simulink library "SimscapeCustomComponents_lib"  (R2025b)
settings: Solver=VariableStepAuto  StartTime=0.0  StopTime=10.0  RelTol=1e-3
undefined symbols (not defined in the file or in its folder): base, baseVdc, capacity, DiscIntNeverNeededParam, ee_sli_rtmsupport, filterInductance, freqeuncy, frequency, gcbh, gflInverter, gfmInverter, iMaxPU, Inertia, initialSOC, plantRating, solar, Ts, ups, Vac, windSystem, windTurbine
libraries: fl_lib x397, nesl_utility x171, eeGeneralControl x85, ee_lib x82, simulink x72, datacenter_lib x68, eeTransforms x38, slpidlib x24, buildingEnergy_lib x20, SimscapeFluids_lib x17, eeSinusoidalMeasurementV2 x8, eePwmGenerator x8
(part 8 of 24)

== system SimscapeCustomComponents_lib/Datacenter/Assemblies/Air Cooled PDU Assembly/PDU Racks ==
  PS Product : fl_lib/Physical Signals/Functions/PS Product
  Server Tray : Subsystem  mask{nGPU=nGPU, gpuTDPperDie=gpuTDPperDie, gpuIdlePower=gpuIdlePower, gpuHBMpower=gpuHBMpower, gpuExponent=gpuExponent, gpuHBMutil=gpuHBMutil, gpuLeakage=gpuLeakage, gpuNominalDieT=gpuNominalDieT, gpuDieThermalC=gpuDieThermalC, gpuHeatSinkR=gpuHeatSinkR, gpuSurfArea=gpuSurfArea, gpuAmbientR=gpuAmbientR, nCPU=nCPU, cpuTDPperSocket=cpuTDPperSocket, cpuIdlePower=cpuIdlePower, cpuExponent=cpuExponent, cpuLeakage=cpuLeakage, cpuNominalDieT=cpuNominalDieT, cpuDieThermalC=cpuDieThermalC, cpuHeatSinkR=cpuHeatSinkR, cpuSurfArea=cpuSurfArea, cpuAmbientR=cpuAmbientR, trayMass=trayMass, trayCp=trayCp, trayThermalR=trayThermalR, initialT=initialT, htc=htc}
      mask prompts: nGPU "Number of GPU (-)"; gpuTDPperDie "GPU TDP per die (W)"; gpuIdlePower "GPU idle power (W)"; gpuHBMpower "HBM power per GPU (W)"; gpuExponent "GPU power utilization exponent (-)"; gpuHBMutil "HBM utilization as fraction of compute utilization (-)"; gpuLeakage "Leakage increase per K above nominal temperature (W/K)"; gpuNominalDieT "Nominal die temperature at TDP (K)"; gpuDieThermalC "GPU die thermal capacitance (J/K)"; gpuHeatSinkR "GPU die-heat-sink thermal resistance (K/W)"; gpuSurfArea "Surface area per die for ambient heat transfer (m^2)"; gpuAmbientR "GPU die-ambient thermal resistance (K/W)"; nCPU "Number of CPU (-)"; cpuTDPperSocket "CPU TDP per socket (W)"; cpuIdlePower "CPU idle power per socket (W)"; cpuExponent "CPU power utilization exponent (-)"; cpuLeakage "Leakage increase per K above nominal temperature (W/K)"; cpuNominalDieT "Nominal die temperature at TDP (K)"; cpuDieThermalC "CPU die thermal capacitance (J/K)"; cpuHeatSinkR "CPU die-heat-sink thermal resistance (K/W)"; cpuSurfArea "Surface area per die for ambient heat transfer (m^2)"; cpuAmbientR "CPU die-ambient thermal resistance (K/W)"; trayMass "Tray mass (kg)"; trayCp "Tray specific heat capacity (J/kg*K)"; trayThermalR "Tray to external thermal resistance (K/W)"; initialT "Initial temperature (K)"; htc "Heat transfer coefficient to ambient (W/m^2.K)"
      settings: CopyFcn=set_param(gcbh,'LinkStatus','none');  PortSchema="{\"entries\":[{\"content\":{\"sides\":[{\"content\":{\"connectorIds\":[\"LConn1\",\"LConn2\",\"LConn3\"]},\"type\":\"ConnectorPlacement.EquallySpacedRectSide\",\"uuid\":\"893f21b9-92d6-433a-96e5-f8193a696c29\"},{\"content\":{\"connectorIds\":[\"RConn1\",\"RConn2\",\"RConn3\"],\"side\":\"RIGHT\"},\"type\":\"ConnectorPlacement.EquallySpacedRectSide\",\"uuid\":\"efd10409-70d8-4a6a-97a2-13f0e6f538e3\"},{\"content\":{\"side\":\"TOP\"},\"type\":\"ConnectorPlacement.EquallySpacedRectSide\",\"uuid\":\"8c9765cd-90e6-46de-916c-606bbb93143e\"},{\"content\":{\"connectorIds\":[\"RConn4\"],\"side\":\"BOTTOM\"},\"type\":\"ConnectorPlacement.EquallySpacedRectSide\",\"uuid\":\"9656b44e-d582-43b0-a7fe-c629821d6c27\"}]},\"type\":\"ConnectorPlacement.EquallySpacedConnector\",\"uuid\":\"add7a682-eb4b-4f46-a5b9-e161ccf96de5\"}],\"packageUris\":[\"http://schema.mathworks.com/mf0/Connector/R2020b\"],\"version\":\"1.0\"}"
      mask Help: web("DocumentationServerTray.html")
      mask DialogControl Container6 Prompt: GPU
      mask DialogControl Container7 Prompt: CPU
      mask DialogControl Container9 Prompt: IT Tray
      mask DialogControl Container8 Prompt: Initial Conditions
      mask Display: image('icon_serverPlate.png');
  TMamb : datacenter_lib/Thermal Multiplier
      settings: InternalSimscapePortConfiguration="{\"Bottom\":[],\"Left\":[{\"id\":\"A\",\"label\":\"A\",\"type\":\"foundation.thermal.thermal\"}],\"Right\":[{\"id\":\"B\",\"label\":\"B\",\"type\":\"foundation.thermal.thermal\"}],\"Top\":[{\"id\":\"Na\",\"label\":\"Na\",\"type\":\"input\"},{\"id\":\"Nb\",\"label\":\"Nb\",\"type\":\"input\"}]}"
  TMcdu : datacenter_lib/Thermal Multiplier
      settings: InternalSimscapePortConfiguration="{\"Bottom\":[],\"Left\":[{\"id\":\"A\",\"label\":\"A\",\"type\":\"foundation.thermal.thermal\"}],\"Right\":[{\"id\":\"B\",\"label\":\"B\",\"type\":\"foundation.thermal.thermal\"}],\"Top\":[{\"id\":\"Na\",\"label\":\"Na\",\"type\":\"input\"},{\"id\":\"Nb\",\"label\":\"Nb\",\"type\":\"input\"}]}"
  nTraysXnRacks : fl_lib/Physical Signals/Sources/PS Constant  constant=nTrays*nRacks
  one : fl_lib/Physical Signals/Sources/PS Constant  constant=1
  U_gpu : PMIOPort  Side=Left
  U_cpu : PMIOPort  Port=2  Side=Left
  Ha : PMIOPort  Port=3  Side=Left
  P : PMIOPort  Port=4  Side=Right
  T_gpu : PMIOPort  Port=5  Side=Right
  T_cpu : PMIOPort  Port=6  Side=Right
  Hc : PMIOPort  Port=7  Side=Right
  connections:
  PS Product/RConn1 -- P/RConn1
  Server Tray/RConn1 -- PS Product/LConn2
  TMamb/LConn3 -- TMcdu/LConn2 -- PS Product/LConn1 -- nTraysXnRacks/RConn1
  Server Tray/LConn3 -- TMamb/RConn1
  Server Tray/RConn4 -- TMcdu/LConn1
  TMamb/LConn2 -- TMcdu/LConn3 -- one/RConn1
  Server Tray/RConn3 -- T_cpu/RConn1
  Server Tray/LConn2 -- U_cpu/RConn1
  TMcdu/RConn1 -- Hc/RConn1
  Server Tray/RConn2 -- T_gpu/RConn1
  TMamb/LConn1 -- Ha/RConn1
  Server Tray/LConn1 -- U_gpu/RConn1

== system SimscapeCustomComponents_lib/Datacenter/Assemblies/Air Cooled PDU Assembly/Rack Air Cooling ==
  Flowrate vs Eff : fl_lib/Physical Signals/Lookup Tables/PS Lookup Table (1D)  x=flowVec m^3/s  f=fanEffVec  interp_method=simscape.enum.interpolation.linear  extrap_method=simscape.enum.extrapolation.nearest
  Flowrate vs Pressure Drop : fl_lib/Physical Signals/Lookup Tables/PS Lookup Table (1D)  x=flowVec m^3/s  f=prDropVec Pa  interp_method=simscape.enum.interpolation.linear  extrap_method=simscape.enum.extrapolation.nearest
  MaxFlowrate : fl_lib/Physical Signals/Functions/PS Gain  gain=max(flowVec) m^3/s
  PS Divide : fl_lib/Physical Signals/Functions/PS Divide
  PS Product : fl_lib/Physical Signals/Functions/PS Product
  PS Product1 : fl_lib/Physical Signals/Functions/PS Product
  PS Saturation : fl_lib/Physical Signals/Nonlinear Operators/PS Saturation  upper_limit=1  lower_limit=0  ZeroCross=true
  Q : Subsystem
  dT : Subsystem
      settings: PortSchema="{\"entries\":[{\"content\":{\"sides\":[{\"content\":{\"connectorIds\":[\"LConn1\"]},\"type\":\"ConnectorPlacement.EquallySpacedRectSide\",\"uuid\":\"24179a54-9ef9-408d-b9e3-71fcbe48c3e7\"},{\"content\":{\"connectorIds\":[\"RConn1\"],\"side\":\"RIGHT\"},\"type\":\"ConnectorPlacement.EquallySpacedRectSide\",\"uuid\":\"9ef8b705-2d29-4693-9aa8-2fb03fb72ba0\"},{\"content\":{\"side\":\"TOP\"},\"type\":\"ConnectorPlacement.EquallySpacedRectSide\",\"uuid\":\"67fd6558-0b74-41b6-9065-c50d20bb7de5\"},{\"content\":{\"connectorIds\":[\"RConn2\"],\"side\":\"BOTTOM\"},\"type\":\"ConnectorPlacement.EquallySpacedRectSide\",\"uuid\":\"dead0843-c913-4c5f-8840-2a92db603c86\"}]},\"type\":\"ConnectorPlacement.EquallySpacedConnector\",\"uuid\":\"734a32c8-d564-4672-86f6-d3d1b9b4eb6d\"}],\"packageUris\":[\"http://schema.mathworks.com/mf0/Connector/R2020b\"],\"version\":\"1.0\"}"
  m_dot_Cp : Subsystem
      settings: PortSchema="{\"entries\":[{\"content\":{\"sides\":[{\"content\":{},\"type\":\"ConnectorPlacement.EquallySpacedRectSide\",\"uuid\":\"30dae9bf-ed85-460d-bbc0-602f54b59459\"},{\"content\":{\"side\":\"RIGHT\"},\"type\":\"ConnectorPlacement.EquallySpacedRectSide\",\"uuid\":\"05907a20-db7b-437b-af9c-28a9e12dbb0f\"},{\"content\":{\"connectorIds\":[\"LConn1\"],\"side\":\"TOP\"},\"type\":\"ConnectorPlacement.EquallySpacedRectSide\",\"uuid\":\"1394250d-0f3a-4d32-aa79-d5be723ed221\"},{\"content\":{\"connectorIds\":[\"RConn1\"],\"side\":\"BOTTOM\"},\"type\":\"ConnectorPlacement.EquallySpacedRectSide\",\"uuid\":\"8d71629e-6ed3-4a45-8875-f0ad6e4187c2\"}]},\"type\":\"ConnectorPlacement.EquallySpacedConnector\",\"uuid\":\"77e9989b-961e-42ca-a28b-c98959ddb965\"}],\"packageUris\":[\"http://schema.mathworks.com/mf0/Connector/R2020b\"],\"version\":\"1.0\"}"
  numFans : fl_lib/Physical Signals/Sources/PS Constant  constant=nFans
  C : PMIOPort  Side=Left
  S : PMIOPort  Port=2  Side=Left
  H : PMIOPort  Port=3  Side=Right
  P : PMIOPort  Port=4  Side=Right
  connections:
  m_dot_Cp/LConn1 -- Q/LConn2
  Q/LConn1 -- dT/RConn2
  dT/LConn1 -- C/RConn1
  H/RConn1 -- dT/RConn1 -- Q/RConn1
  PS Product/LConn1 -- Flowrate vs Pressure Drop/RConn1
  numFans/RConn1 -- PS Product1/LConn1
  PS Saturation/RConn1 -- MaxFlowrate/LConn1
  PS Divide/RConn1 -- P/RConn1
  PS Divide/LConn2 -- Flowrate vs Eff/RConn1
  PS Product1/RConn1 -- PS Divide/LConn1
  PS Saturation/LConn1 -- S/RConn1
  PS Product1/LConn2 -- PS Product/RConn1
  m_dot_Cp/RConn1 -- MaxFlowrate/RConn1 -- Flowrate vs Pressure Drop/LConn1 -- PS Product/LConn2 -- Flowrate vs Eff/LConn1

== system SimscapeCustomComponents_lib/Datacenter/Assemblies/PDU + CDU Assembly (LUT)/CDU (LUT) ==
  Capacity vs. Flowrate : fl_lib/Physical Signals/Lookup Tables/PS Lookup Table (1D)  x=flowrate_vec m^3/s  f=capacity_vec W  interp_method=simscape.enum.interpolation.linear  extrap_method=simscape.enum.extrapolation.nearest
  Controlled Heat Flow Rate Source : fl_lib/Thermal/Thermal Sources/Controlled Heat Flow Rate Source
  Electric Power : fl_lib/Physical Signals/Functions/PS Divide
  PS Product : fl_lib/Physical Signals/Functions/PS Product
  PS Product1 : fl_lib/Physical Signals/Functions/PS Product
  Pressure Drop vs. Num Pump & Flowrate : fl_lib/Physical Signals/Lookup Tables/PS Lookup Table (2D)  x1=flowrate_vec m^3/s  x2=1:numPump  f=prDrop_mat Pa  interp_method=simscape.enum.interpolation.linear  extrap_method=simscape.enum.extrapolation.nearest
  Pump Eff. vs. Flowrate : fl_lib/Physical Signals/Lookup Tables/PS Lookup Table (1D)  x=flowrate_vec m^3/s  f=effPump_vec  interp_method=simscape.enum.interpolation.linear  extrap_method=simscape.enum.extrapolation.nearest
  Thermal Reference : fl_lib/Thermal/Thermal Elements/Thermal Reference
  flowrate : Subsystem
  S : PMIOPort  Side=Left
  N : PMIOPort  Port=2  Side=Left
  H : PMIOPort  Port=3  Side=Left
  P : PMIOPort  Port=4  Side=Right
  Q : PMIOPort  Port=5  Side=Right
  connections:
  S/RConn1 -- flowrate/LConn1
  Capacity vs. Flowrate/LConn1 -- flowrate/RConn1 -- PS Product/LConn2 -- Pump Eff. vs. Flowrate/LConn1 -- Pressure Drop vs. Num Pump & Flowrate/LConn1
  Controlled Heat Flow Rate Source/RConn1 -- Q/RConn1 -- PS Product1/RConn1
  Capacity vs. Flowrate/RConn1 -- PS Product1/LConn1
  Controlled Heat Flow Rate Source/RConn2 -- H/RConn1
  Electric Power/LConn1 -- PS Product/RConn1
  Electric Power/RConn1 -- P/RConn1
  PS Product/LConn1 -- Pressure Drop vs. Num Pump & Flowrate/RConn1
  N/RConn1 -- Pressure Drop vs. Num Pump & Flowrate/LConn2 -- PS Product1/LConn2
  Controlled Heat Flow Rate Source/LConn1 -- Thermal Reference/LConn1
  Electric Power/LConn2 -- Pump Eff. vs. Flowrate/RConn1

== system SimscapeCustomComponents_lib/Datacenter/Assemblies/PDU + CDU Assembly (LUT)/PDU Racks ==
  PS Product : fl_lib/Physical Signals/Functions/PS Product
  Server Tray : Subsystem  mask{nGPU=nGPU, gpuTDPperDie=gpuTDPperDie, gpuIdlePower=gpuIdlePower, gpuHBMpower=gpuHBMpower, gpuExponent=gpuExponent, gpuHBMutil=gpuHBMutil, gpuLeakage=gpuLeakage, gpuNominalDieT=gpuLeakage, gpuDieThermalC=gpuDieThermalC, gpuHeatSinkR=gpuHeatSinkR, gpuSurfArea=gpuSurfArea, gpuAmbientR=gpuAmbientR, nCPU=nCPU, cpuTDPperSocket=cpuTDPperSocket, cpuIdlePower=cpuIdlePower, cpuExponent=cpuExponent, cpuLeakage=cpuLeakage, cpuNominalDieT=cpuNominalDieT, cpuDieThermalC=cpuDieThermalC, cpuHeatSinkR=cpuHeatSinkR, cpuSurfArea=cpuSurfArea, cpuAmbientR=cpuAmbientR, trayMass=trayMass, trayCp=trayCp, trayThermalR=trayThermalR, initialT=initialT, htc=htc}
      mask prompts: nGPU "Number of GPU (-)"; gpuTDPperDie "GPU TDP per die (W)"; gpuIdlePower "GPU idle power (W)"; gpuHBMpower "HBM power per GPU (W)"; gpuExponent "GPU power utilization exponent (-)"; gpuHBMutil "HBM utilization as fraction of compute utilization (-)"; gpuLeakage "Leakage increase per K above nominal temperature (W/K)"; gpuNominalDieT "Nominal die temperature at TDP (K)"; gpuDieThermalC "GPU die thermal capacitance (J/K)"; gpuHeatSinkR "GPU die-heat-sink thermal resistance (K/W)"; gpuSurfArea "Surface area per die for ambient heat transfer (m^2)"; gpuAmbientR "GPU die-ambient thermal resistance (K/W)"; nCPU "Number of CPU (-)"; cpuTDPperSocket "CPU TDP per socket (W)"; cpuIdlePower "CPU idle power per socket (W)"; cpuExponent "CPU power utilization exponent (-)"; cpuLeakage "Leakage increase per K above nominal temperature (W/K)"; cpuNominalDieT "Nominal die temperature at TDP (K)"; cpuDieThermalC "CPU die thermal capacitance (J/K)"; cpuHeatSinkR "CPU die-heat-sink thermal resistance (K/W)"; cpuSurfArea "Surface area per die for ambient heat transfer (m^2)"; cpuAmbientR "CPU die-ambient thermal resistance (K/W)"; trayMass "Tray mass (kg)"; trayCp "Tray specific heat capacity (J/kg*K)"; trayThermalR "Tray to external thermal resistance (K/W)"; initialT "Initial temperature (K)"; htc "Heat transfer coefficient to ambient (W/m^2.K)"
      settings: CopyFcn=set_param(gcbh,'LinkStatus','none');  PortSchema="{\"entries\":[{\"content\":{\"sides\":[{\"content\":{\"connectorIds\":[\"LConn1\",\"LConn2\",\"LConn3\"]},\"type\":\"ConnectorPlacement.EquallySpacedRectSide\",\"uuid\":\"893f21b9-92d6-433a-96e5-f8193a696c29\"},{\"content\":{\"connectorIds\":[\"RConn1\",\"RConn2\",\"RConn3\"],\"side\":\"RIGHT\"},\"type\":\"ConnectorPlacement.EquallySpacedRectSide\",\"uuid\":\"efd10409-70d8-4a6a-97a2-13f0e6f538e3\"},{\"content\":{\"side\":\"TOP\"},\"type\":\"ConnectorPlacement.EquallySpacedRectSide\",\"uuid\":\"8c9765cd-90e6-46de-916c-606bbb93143e\"},{\"content\":{\"connectorIds\":[\"RConn4\"],\"side\":\"BOTTOM\"},\"type\":\"ConnectorPlacement.EquallySpacedRectSide\",\"uuid\":\"9656b44e-d582-43b0-a7fe-c629821d6c27\"}]},\"type\":\"ConnectorPlacement.EquallySpacedConnector\",\"uuid\":\"add7a682-eb4b-4f46-a5b9-e161ccf96de5\"}],\"packageUris\":[\"http://schema.mathworks.com/mf0/Connector/R2020b\"],\"version\":\"1.0\"}"
      mask Help: web("DocumentationServerTray.html")
      mask DialogControl Container6 Prompt: GPU
      mask DialogControl Container7 Prompt: CPU
      mask DialogControl Container9 Prompt: IT Tray
      mask DialogControl Container8 Prompt: Initial Conditions
      mask Display: image('icon_serverPlate.png');
  TMamb : datacenter_lib/Thermal Multiplier
      settings: InternalSimscapePortConfiguration="{\"Bottom\":[],\"Left\":[{\"id\":\"A\",\"label\":\"A\",\"type\":\"foundation.thermal.thermal\"}],\"Right\":[{\"id\":\"B\",\"label\":\"B\",\"type\":\"foundation.thermal.thermal\"}],\"Top\":[{\"id\":\"Na\",\"label\":\"Na\",\"type\":\"input\"},{\"id\":\"Nb\",\"label\":\"Nb\",\"type\":\"input\"}]}"
  TMcdu : datacenter_lib/Thermal Multiplier
      settings: InternalSimscapePortConfiguration="{\"Bottom\":[],\"Left\":[{\"id\":\"A\",\"label\":\"A\",\"type\":\"foundation.thermal.thermal\"}],\"Right\":[{\"id\":\"B\",\"label\":\"B\",\"type\":\"foundation.thermal.thermal\"}],\"Top\":[{\"id\":\"Na\",\"label\":\"Na\",\"type\":\"input\"},{\"id\":\"Nb\",\"label\":\"Nb\",\"type\":\"input\"}]}"
  nTraysXnRacks : fl_lib/Physical Signals/Sources/PS Constant  constant=nTrays*nRacks
  one : fl_lib/Physical Signals/Sources/PS Constant  constant=1
  U_gpu : PMIOPort  Side=Left
  U_cpu : PMIOPort  Port=2  Side=Left
  Ha : PMIOPort  Port=3  Side=Left
  P : PMIOPort  Port=4  Side=Right
  T_gpu : PMIOPort  Port=5  Side=Right
  T_cpu : PMIOPort  Port=6  Side=Right
  Hc : PMIOPort  Port=7  Side=Right
  connections:
  PS Product/RConn1 -- P/RConn1
  Server Tray/RConn1 -- PS Product/LConn2
  TMamb/LConn3 -- TMcdu/LConn2 -- PS Product/LConn1 -- nTraysXnRacks/RConn1
  Server Tray/LConn3 -- TMamb/RConn1
  Server Tray/RConn4 -- TMcdu/LConn1
  TMamb/LConn2 -- TMcdu/LConn3 -- one/RConn1
  Server Tray/RConn3 -- T_cpu/RConn1
  Server Tray/LConn2 -- U_cpu/RConn1
  TMcdu/RConn1 -- Hc/RConn1
  Server Tray/RConn2 -- T_gpu/RConn1
  TMamb/LConn1 -- Ha/RConn1
  Server Tray/LConn1 -- U_gpu/RConn1

== system SimscapeCustomComponents_lib/Datacenter/Assemblies/PDU + CDU Assembly (TL)/CDU (TL) ==
  CDU Pipe : fl_lib/Thermal Liquid/Elements/Pipe (TL)  length=effPipeLen m  area=intFluidPipeArea m^2  Dh=sqrt(4*intFluidPipeArea/pi) m  length_add=1e-2 m  roughness=15e-6 m  Re_lam=2000  Re_tur=4000  shape_factor=64  Nu_lam=3.66  dynamic_compressibility=true  inertia=false  p0=iniP MPa  T0=iniT K  mdot0=0 kg/s  p_nominal=0.101325 MPa  T_nominal=293.15 K
  Centrifugal Pump (TL) : SimscapeFluids_lib/Thermal Liquid/Pumps & Motors/Centrifugal Pump (TL)  pump_parameterization=fluids.thermal_liquid.pumps_motors.enum.CentrifugalPumpParameterization.Table1D  capacity_ref_nominal=45 lpm  head_ref_nominal=40 m  power_ref_nominal=0.85 kW  head_ref_max=60 m  capacity_ref_max=80 lpm  omega_ref_analytic=1770 rpm  flow_rate_1D_TLU=pumpCapacityVec m^3/s  head_1D_TLU=pumpRefHeadVec m  power_1D_TLU=pumpRefBrkPowVec kW  omega_ref_1D=pumpNominalRPM rpm  rho_ref_1D=refDensity kg/m^3  omega_threshold_factor=1e-2  flow_rate_2D_TLU=[16.67, 23.33, 30, 40, 53.33, 60] lpm  omega_2D_TLU=[2450, 2800, 3150, 3500] rpm  head_2D_TLU=[25, 32.7, 42.5, 50; 24, 31.7, 41, 49; 22.7, 30.5, 39, 47.5; 20, 28, 36, 45; 15.7, 24, 32, 40; 12.5, 21, 29.5, 37.5] m  power_2D_TLU=[.28, .38, .5, .6; .31, .41, .55, .68; .33, .44, .6, .75; .36, .48, .65, .83; .38, .53, .72, .93; .39, .55, .75, .97] kW  rho_ref_2D=998.21 kg/m^3  diameter_ratio=pumpImpellerDiaFactor  mech_orientation=fluids.thermal_liquid.pumps_motors.enum.CentrifugalPumpMechOrientation.Positive  area=intFluidPipeArea/nPumps m^2  operation_check=simscape.enum.assert.action.none
      settings: InternalSimscapePortConfiguration="{\"Bottom\":[],\"Left\":[{\"id\":\"A\",\"label\":\"A\",\"type\":\"foundation.thermal_liquid.thermal_liquid\"},{\"id\":\"B\",\"label\":\"B\",\"type\":\"foundation.thermal_liquid.thermal_liquid\"}],\"Right\":[{\"id\":\"R\",\"label\":\"R\",\"type\":\"foundation.mechanical.rotational.rotational\"},{\"id\":\"C\",\"label\":\"C\",\"type\":\"foundation.mechanical.rotational.rotational\"}],\"Top\":[]}"
  Expansion Tank : SimscapeFluids_lib/Thermal Liquid/Tanks & Accumulators/Gas-Charged Accumulator (TL)  capacity=intFluidVol m^3  dead_volume=1e-3 m^3  p_precharge_gauge=iniP MPa  k_sh=1.4  area=intFluidPipeArea m^2  stiff_coeff=1e4 MPa/m^3  damping_coeff=1e4 MPa*s/m^6  liquid_volume_specify=on  liquid_volume_priority=None  liquid_volume=5e-3 m^3  liquid_volume_nominal_specify=off  liquid_volume_nominal_value=1  liquid_volume_nominal_unit=m^3  liquid_mass_specify=off  liquid_mass_priority=None  liquid_mass=5 kg  liquid_mass_nominal_specify=off  liquid_mass_nominal_value=1  liquid_mass_nominal_unit=kg  p_I_specify=on  p_I_priority=High  p_I=4*iniP MPa  p_I_nominal_specify=off  p_I_nominal_value=1  p_I_nominal_unit=MPa  T_I_specify=on  T_I_priority=High  T_I=iniT K  T_I_nominal_specify=off  T_I_nominal_value=1  T_I_nominal_unit=K
      settings: InternalSimscapePortConfiguration="{\"Bottom\":[],\"Left\":[],\"Right\":[{\"id\":\"A\",\"label\":\"A\",\"type\":\"foundation.thermal_liquid.thermal_liquid\"},{\"id\":\"H\",\"label\":\"H\",\"type\":\"foundation.thermal.thermal\"}],\"Top\":[]}"
  Flow Multiplier : datacenter_lib/Flow Multiplier
      settings: InternalSimscapePortConfiguration="{\"Bottom\":[],\"Left\":[{\"id\":\"A\",\"label\":\"A\",\"type\":\"foundation.thermal_liquid.thermal_liquid\"}],\"Right\":[{\"id\":\"B\",\"label\":\"B\",\"type\":\"foundation.thermal_liquid.thermal_liquid\"}],\"Top\":[{\"id\":\"Na\",\"label\":\"Na\",\"type\":\"input\"},{\"id\":\"Nb\",\"label\":\"Nb\",\"type\":\"input\"}]}"
  "Flow Multiplier " : datacenter_lib/Flow Multiplier
      settings: InternalSimscapePortConfiguration="{\"Bottom\":[],\"Left\":[{\"id\":\"A\",\"label\":\"A\",\"type\":\"foundation.thermal_liquid.thermal_liquid\"}],\"Right\":[{\"id\":\"B\",\"label\":\"B\",\"type\":\"foundation.thermal_liquid.thermal_liquid\"}],\"Top\":[{\"id\":\"Na\",\"label\":\"Na\",\"type\":\"input\"},{\"id\":\"Nb\",\"label\":\"Nb\",\"type\":\"input\"}]}"
  Flow Rate Sensor (TL) : fl_lib/Thermal Liquid/Sensors/Flow Rate Sensor (TL)  mass_flow_measure=false  volumetric_flow_measure=true  energy_flow_measure=false
      settings: InternalSimscapePortConfiguration="{\"Bottom\":[],\"Left\":[{\"id\":\"A\",\"label\":\"A\",\"type\":\"foundation.thermal_liquid.thermal_liquid\"}],\"Right\":[{\"id\":\"B\",\"label\":\"B\",\"type\":\"foundation.thermal_liquid.thermal_liquid\"},{\"id\":\"V\",\"label\":\"V\",\"type\":\"output\"}],\"Top\":[]}"
  Flow Resistance (TL) : fl_lib/Thermal Liquid/Elements/Flow Resistance (TL)  delta_p_nominal=0.1*min(intFluidPrDrop) kPa  mdot_nominal=min(intFluidMdot) kg/s  area=intFluidPipeArea m^2  laminar_fraction=1e-3
  "Flow Resistance (TL) " : fl_lib/Thermal Liquid/Elements/Flow Resistance (TL)  delta_p_nominal=0.1*min(intFluidPrDrop) kPa  mdot_nominal=min(intFluidMdot) kg/s  area=intFluidPipeArea m^2  laminar_fraction=1e-3
  InternalFluid : SimscapeFluids_lib/Thermal Liquid/Utilities/Thermal Liquid Properties (TL)  fluid_list=fluids.thermal_liquid.utilities.enum.thermal_liquid_fluid_list.water  concentration_param_EG=fluids.thermal_liquid.utilities.enum.thermal_liquid_concentration.volume_fraction  concentration_param_PG=fluids.thermal_liquid.utilities.enum.thermal_liquid_concentration.volume_fraction  c_mass_SW=3.5e-3  c_mass_EG=0.1  c_mass_PG=0.1  c_mass_GL=0.1  c_vol_EG=0.1  c_vol_PG=0.1  beta_const_EG=2.1791 GPa  beta_const_PG=2.1791 GPa  beta_const_GL=2.1791 GPa  p_min_EG=0.01 MPa  p_min_PG=0.01 MPa  p_min_GL=0.01 MPa  p_max_EG=50 MPa  p_max_PG=50 MPa  p_max_GL=50 MPa  p_atm=0.101325 MPa  properties_range_check=simscape.enum.assert.action.error
  One : fl_lib/Physical Signals/Sources/PS Constant  constant=1
  PS Saturation : fl_lib/Physical Signals/Nonlinear Operators/PS Saturation  upper_limit=speedLimFactor  lower_limit=0  ZeroCross=true
  Perfect Insulator1 : fl_lib/Thermal/Thermal Elements/Perfect Insulator  T_specify=off  T_priority=None  T=293.15 K  T_nominal_specify=off  T_nominal_value=1  T_nominal_unit=K
  Pressure & Temperature Sensor (TL) : fl_lib/Thermal Liquid/Sensors/Pressure & Temperature Sensor (TL)  reference=foundation.enum.MeasurementReference.difference  pressure=true  pressure_spec=foundation.enum.PressureMeasementSpec.Absolute  temperature=false
      settings: InternalSimscapePortConfiguration="{\"Bottom\":[],\"Left\":[{\"id\":\"A\",\"label\":\"A\",\"type\":\"foundation.thermal_liquid.thermal_liquid\"}],\"Right\":[{\"id\":\"B\",\"label\":\"B\",\"type\":\"foundation.thermal_liquid.thermal_liquid\"},{\"id\":\"P\",\"label\":\"P\",\"type\":\"output\"}],\"Top\":[]}"
  Pump Efficiency : Subsystem
      settings: PortSchema="{\"entries\":[{\"content\":{\"sides\":[{\"content\":{\"connectorIds\":[\"LConn1\"]},\"type\":\"ConnectorPlacement.EquallySpacedRectSide\",\"uuid\":\"7c880f53-79d7-4fc1-b853-6a19eeb267d6\"},{\"content\":{\"connectorIds\":[\"RConn1\"],\"side\":\"RIGHT\"},\"type\":\"ConnectorPlacement.EquallySpacedRectSide\",\"uuid\":\"ee796b5d-8f71-4c2c-8982-d65c9b09dfff\"},{\"content\":{\"connectorIds\":[\"LConn2\",\"LConn3\"],\"side\":\"TOP\"},\"type\":\"ConnectorPlacement.EquallySpacedRectSide\",\"uuid\":\"11e8f51e-a30e-473a-bd43-abeec225f5c9\"}]},\"type\":\"ConnectorPlacement.EquallySpacedConnector\",\"uuid\":\"3106b96b-5b56-4bfa-809a-5c3e3f25fbb5\"}],\"packageUris\":[\"http://schema.mathworks.com/mf0/Connector/R2020b\"],\"version\":\"1.0\"}"
  Pump Nominal Rating : fl_lib/Physical Signals/Functions/PS Gain  gain=pumpNominalRPM rpm
  Specific Dissipation Heat Exchanger (TL-TL) : SimscapeFluids_lib/Heat Exchangers/Thermal Liquid/Specific Dissipation Heat Exchanger (TL-TL)  mdot1_TLU=intFluidMdot kg/s  mdot2_TLU=extFluidMdot kg/s  SD_TLU=spDissipationTbl kW/K  Q_check=simscape.enum.assert.action.none  mdot_dp_TLU_1=intFluidMdot kg/s  p_diff_TLU_1=intFluidPrDrop-0.2*min(intFluidPrDrop) kPa  T_ref_in_1=refT K  p_ref_in_1=refP MPa  mdot_threshold_1=1e-3 kg/s  liquid_volume_1=intFluidVol m^3  area_1=intFluidPipeArea m^2  mdot_dp_TLU_2=extFluidMdot kg/s  p_diff_TLU_2=extFluidPrDrop kPa  T_ref_in_2=refT K  p_ref_in_2=refP MPa  mdot_threshold_2=1e-3 kg/s  liquid_volume_2=extFluidVol m^3  area_2=extFluidPipeArea m^2  dynamic_compressibility_1=true  T0_1=iniT K  p0_1=iniP MPa  T_nominal_1=293.15 K  p_nominal_1=0.101325 MPa  dynamic_compressibility_2=true  T0_2=iniT K  p0_2=iniP MPa  T_nominal_2=293.15 K  p_nominal_2=0.101325 MPa
      settings: InternalSimscapePortConfiguration="{\"Bottom\":[],\"Left\":[{\"id\":\"A1\",\"label\":\"A1\",\"type\":\"foundation.thermal_liquid.thermal_liquid\"},{\"id\":\"B1\",\"label\":\"B1\",\"type\":\"foundation.thermal_liquid.thermal_liquid\"}],\"Right\":[{\"id\":\"A2\",\"label\":\"A2\",\"type\":\"foundation.thermal_liquid.thermal_liquid\"},{\"id\":\"B2\",\"label\":\"B2\",\"type\":\"foundation.thermal_liquid.thermal_liquid\"}],\"Top\":[]}"
  Subsystem : Subsystem
  numPump : fl_lib/Physical Signals/Nonlinear Operators/PS Saturation  upper_limit=nPumps  lower_limit=0  ZeroCross=true
  S : PMIOPort  Side=Left
  N : PMIOPort  Port=2  Side=Left
  Ae : PMIOPort  Port=3  Side=Left
  H : PMIOPort  Port=4  Side=Left
  P : PMIOPort  Port=5  Side=Right
  Be : PMIOPort  Port=6  Side=Right
  connections:
  One/RConn1 -- "Flow Multiplier "/LConn3 -- Flow Multiplier/LConn2
  numPump/RConn1 -- "Flow Multiplier "/LConn2 -- Pump Efficiency/LConn3 -- Flow Multiplier/LConn3
  Flow Rate Sensor (TL)/RConn1 -- "Flow Multiplier "/RConn1
  Centrifugal Pump (TL)/LConn2 -- "Flow Multiplier "/LConn1
  N/RConn1 -- numPump/LConn1
  Pump Efficiency/LConn1 -- Pressure & Temperature Sensor (TL)/RConn2
  Flow Rate Sensor (TL)/RConn2 -- Pump Efficiency/LConn2
  P/RConn1 -- Pump Efficiency/RConn1
  Pressure & Temperature Sensor (TL)/RConn1 -- "Flow Resistance (TL) "/LConn1 -- Flow Rate Sensor (TL)/LConn1
  Flow Multiplier/RConn1 -- Centrifugal Pump (TL)/LConn1
  Flow Multiplier/LConn1 -- CDU Pipe/RConn1 -- Pressure & Temperature Sensor (TL)/LConn1
  "Flow Resistance (TL) "/RConn1 -- Specific Dissipation Heat Exchanger (TL-TL)/LConn1
  PS Saturation/LConn1 -- S/RConn1
  Pump Nominal Rating/LConn1 -- PS Saturation/RConn1
  Perfect Insulator1/LConn1 -- Expansion Tank/RConn2
  Pump Nominal Rating/RConn1 -- Subsystem/RConn1
  Centrifugal Pump (TL)/RConn1 -- Subsystem/LConn1
  Centrifugal Pump (TL)/RConn2 -- Subsystem/LConn2
  Flow Resistance (TL)/RConn1 -- Specific Dissipation Heat Exchanger (TL-TL)/LConn2 -- InternalFluid/RConn1
  Specific Dissipation Heat Exchanger (TL-TL)/RConn1 -- Ae/RConn1
  Flow Resistance (TL)/LConn1 -- CDU Pipe/LConn1 -- Expansion Tank/RConn1
  Specific Dissipation Heat Exchanger (TL-TL)/RConn2 -- Be/RConn1
  H/RConn1 -- CDU Pipe/LConn2

== system SimscapeCustomComponents_lib/Datacenter/Assemblies/PDU + CDU Assembly (TL)/PDU Racks ==
  PS Product : fl_lib/Physical Signals/Functions/PS Product
  Server Tray : Subsystem  mask{nGPU=nGPU, gpuTDPperDie=gpuTDPperDie, gpuIdlePower=gpuIdlePower, gpuHBMpower=gpuHBMpower, gpuExponent=gpuExponent, gpuHBMutil=gpuHBMutil, gpuLeakage=gpuLeakage, gpuNominalDieT=gpuLeakage, gpuDieThermalC=gpuDieThermalC, gpuHeatSinkR=gpuHeatSinkR, gpuSurfArea=gpuSurfArea, gpuAmbientR=gpuAmbientR, nCPU=nCPU, cpuTDPperSocket=cpuTDPperSocket, cpuIdlePower=cpuIdlePower, cpuExponent=cpuExponent, cpuLeakage=cpuLeakage, cpuNominalDieT=cpuNominalDieT, cpuDieThermalC=cpuDieThermalC, cpuHeatSinkR=cpuHeatSinkR, cpuSurfArea=cpuSurfArea, cpuAmbientR=cpuAmbientR, trayMass=trayMass, trayCp=trayCp, trayThermalR=trayThermalR, initialT=initialT, htc=htc}
      mask prompts: nGPU "Number of GPU (-)"; gpuTDPperDie "GPU TDP per die (W)"; gpuIdlePower "GPU idle power (W)"; gpuHBMpower "HBM power per GPU (W)"; gpuExponent "GPU power utilization exponent (-)"; gpuHBMutil "HBM utilization as fraction of compute utilization (-)"; gpuLeakage "Leakage increase per K above nominal temperature (W/K)"; gpuNominalDieT "Nominal die temperature at TDP (K)"; gpuDieThermalC "GPU die thermal capacitance (J/K)"; gpuHeatSinkR "GPU die-heat-sink thermal resistance (K/W)"; gpuSurfArea "Surface area per die for ambient heat transfer (m^2)"; gpuAmbientR "GPU die-ambient thermal resistance (K/W)"; nCPU "Number of CPU (-)"; cpuTDPperSocket "CPU TDP per socket (W)"; cpuIdlePower "CPU idle power per socket (W)"; cpuExponent "CPU power utilization exponent (-)"; cpuLeakage "Leakage increase per K above nominal temperature (W/K)"; cpuNominalDieT "Nominal die temperature at TDP (K)"; cpuDieThermalC "CPU die thermal capacitance (J/K)"; cpuHeatSinkR "CPU die-heat-sink thermal resistance (K/W)"; cpuSurfArea "Surface area per die for ambient heat transfer (m^2)"; cpuAmbientR "CPU die-ambient thermal resistance (K/W)"; trayMass "Tray mass (kg)"; trayCp "Tray specific heat capacity (J/kg*K)"; trayThermalR "Tray to external thermal resistance (K/W)"; initialT "Initial temperature (K)"; htc "Heat transfer coefficient to ambient (W/m^2.K)"
      settings: CopyFcn=set_param(gcbh,'LinkStatus','none');  PortSchema="{\"entries\":[{\"content\":{\"sides\":[{\"content\":{\"connectorIds\":[\"LConn1\",\"LConn2\",\"LConn3\"]},\"type\":\"ConnectorPlacement.EquallySpacedRectSide\",\"uuid\":\"893f21b9-92d6-433a-96e5-f8193a696c29\"},{\"content\":{\"connectorIds\":[\"RConn1\",\"RConn2\",\"RConn3\"],\"side\":\"RIGHT\"},\"type\":\"ConnectorPlacement.EquallySpacedRectSide\",\"uuid\":\"efd10409-70d8-4a6a-97a2-13f0e6f538e3\"},{\"content\":{\"side\":\"TOP\"},\"type\":\"ConnectorPlacement.EquallySpacedRectSide\",\"uuid\":\"8c9765cd-90e6-46de-916c-606bbb93143e\"},{\"content\":{\"connectorIds\":[\"RConn4\"],\"side\":\"BOTTOM\"},\"type\":\"ConnectorPlacement.EquallySpacedRectSide\",\"uuid\":\"9656b44e-d582-43b0-a7fe-c629821d6c27\"}]},\"type\":\"ConnectorPlacement.EquallySpacedConnector\",\"uuid\":\"add7a682-eb4b-4f46-a5b9-e161ccf96de5\"}],\"packageUris\":[\"http://schema.mathworks.com/mf0/Connector/R2020b\"],\"version\":\"1.0\"}"
      mask Help: web("DocumentationServerTray.html")
      mask DialogControl Container6 Prompt: GPU
      mask DialogControl Container7 Prompt: CPU
      mask DialogControl Container9 Prompt: IT Tray
      mask DialogControl Container8 Prompt: Initial Conditions
      mask Display: image('icon_serverPlate.png');
  TMamb : datacenter_lib/Thermal Multiplier
      settings: InternalSimscapePortConfiguration="{\"Bottom\":[],\"Left\":[{\"id\":\"A\",\"label\":\"A\",\"type\":\"foundation.thermal.thermal\"}],\"Right\":[{\"id\":\"B\",\"label\":\"B\",\"type\":\"foundation.thermal.thermal\"}],\"Top\":[{\"id\":\"Na\",\"label\":\"Na\",\"type\":\"input\"},{\"id\":\"Nb\",\"label\":\"Nb\",\"type\":\"input\"}]}"
  TMcdu : datacenter_lib/Thermal Multiplier
      settings: InternalSimscapePortConfiguration="{\"Bottom\":[],\"Left\":[{\"id\":\"A\",\"label\":\"A\",\"type\":\"foundation.thermal.thermal\"}],\"Right\":[{\"id\":\"B\",\"label\":\"B\",\"type\":\"foundation.thermal.thermal\"}],\"Top\":[{\"id\":\"Na\",\"label\":\"Na\",\"type\":\"input\"},{\"id\":\"Nb\",\"label\":\"Nb\",\"type\":\"input\"}]}"
  nTraysXnRacks : fl_lib/Physical Signals/Sources/PS Constant  constant=nTrays*nRacks
  one : fl_lib/Physical Signals/Sources/PS Constant  constant=1
  U_gpu : PMIOPort  Side=Left
  U_cpu : PMIOPort  Port=2  Side=Left
  Ha : PMIOPort  Port=3  Side=Left
  P : PMIOPort  Port=4  Side=Right
  T_gpu : PMIOPort  Port=5  Side=Right
  T_cpu : PMIOPort  Port=6  Side=Right
  Hc : PMIOPort  Port=7  Side=Right
  connections:
  PS Product/RConn1 -- P/RConn1
  Server Tray/RConn1 -- PS Product/LConn2
  TMamb/LConn3 -- TMcdu/LConn2 -- PS Product/LConn1 -- nTraysXnRacks/RConn1
  Server Tray/LConn3 -- TMamb/RConn1
  Server Tray/RConn4 -- TMcdu/LConn1
  TMamb/LConn2 -- TMcdu/LConn3 -- one/RConn1
  Server Tray/RConn3 -- T_cpu/RConn1
  Server Tray/LConn2 -- U_cpu/RConn1
  TMcdu/RConn1 -- Hc/RConn1
  Server Tray/RConn2 -- T_gpu/RConn1
  TMamb/LConn1 -- Ha/RConn1
  Server Tray/LConn1 -- U_gpu/RConn1

== system SimscapeCustomComponents_lib/Datacenter/Assemblies/PDU + CDU Assembly (TL-TL)/CDU (TL) Detailed ==
  Centrifugal Pump (TL) : SimscapeFluids_lib/Thermal Liquid/Pumps & Motors/Centrifugal Pump (TL)  pump_parameterization=fluids.thermal_liquid.pumps_motors.enum.CentrifugalPumpParameterization.Table1D  capacity_ref_nominal=45 lpm  head_ref_nominal=40 m  power_ref_nominal=0.85 kW  head_ref_max=60 m  capacity_ref_max=80 lpm  omega_ref_analytic=1770 rpm  flow_rate_1D_TLU=pumpCapacityVec m^3/s  head_1D_TLU=pumpRefHeadVec m  power_1D_TLU=pumpRefBrkPowVec kW  omega_ref_1D=pumpNominalRPM rpm  rho_ref_1D=refDensity kg/m^3  omega_threshold_factor=1e-2  flow_rate_2D_TLU=[16.67, 23.33, 30, 40, 53.33, 60] lpm  omega_2D_TLU=[2450, 2800, 3150, 3500] rpm  head_2D_TLU=[25, 32.7, 42.5, 50; 24, 31.7, 41, 49; 22.7, 30.5, 39, 47.5; 20, 28, 36, 45; 15.7, 24, 32, 40; 12.5, 21, 29.5, 37.5] m  power_2D_TLU=[.28, .38, .5, .6; .31, .41, .55, .68; .33, .44, .6, .75; .36, .48, .65, .83; .38, .53, .72, .93; .39, .55, .75, .97] kW  rho_ref_2D=998.21 kg/m^3  diameter_ratio=pumpImpellerDiaFactor  mech_orientation=fluids.thermal_liquid.pumps_motors.enum.CentrifugalPumpMechOrientation.Positive  area=intFluidPipeArea/nPumps m^2  operation_check=simscape.enum.assert.action.none
      settings: InternalSimscapePortConfiguration="{\"Bottom\":[],\"Left\":[{\"id\":\"A\",\"label\":\"A\",\"type\":\"foundation.thermal_liquid.thermal_liquid\"},{\"id\":\"B\",\"label\":\"B\",\"type\":\"foundation.thermal_liquid.thermal_liquid\"}],\"Right\":[{\"id\":\"R\",\"label\":\"R\",\"type\":\"foundation.mechanical.rotational.rotational\"},{\"id\":\"C\",\"label\":\"C\",\"type\":\"foundation.mechanical.rotational.rotational\"}],\"Top\":[]}"
  Expansion Tank : SimscapeFluids_lib/Thermal Liquid/Tanks & Accumulators/Gas-Charged Accumulator (TL)  capacity=intFluidVol m^3  dead_volume=1e-3 m^3  p_precharge_gauge=iniP MPa  k_sh=1.4  area=intFluidPipeArea m^2  stiff_coeff=1e4 MPa/m^3  damping_coeff=1e4 MPa*s/m^6  liquid_volume_specify=on  liquid_volume_priority=None  liquid_volume=5e-3 m^3  liquid_volume_nominal_specify=off  liquid_volume_nominal_value=1  liquid_volume_nominal_unit=m^3  liquid_mass_specify=off  liquid_mass_priority=None  liquid_mass=5 kg  liquid_mass_nominal_specify=off  liquid_mass_nominal_value=1  liquid_mass_nominal_unit=kg  p_I_specify=on  p_I_priority=High  p_I=4*iniP MPa  p_I_nominal_specify=off  p_I_nominal_value=1  p_I_nominal_unit=MPa  T_I_specify=on  T_I_priority=High  T_I=iniT K  T_I_nominal_specify=off  T_I_nominal_value=1  T_I_nominal_unit=K
      settings: InternalSimscapePortConfiguration="{\"Bottom\":[],\"Left\":[],\"Right\":[{\"id\":\"A\",\"label\":\"A\",\"type\":\"foundation.thermal_liquid.thermal_liquid\"},{\"id\":\"H\",\"label\":\"H\",\"type\":\"foundation.thermal.thermal\"}],\"Top\":[]}"
  Flow Multiplier : datacenter_lib/Flow Multiplier
      settings: InternalSimscapePortConfiguration="{\"Bottom\":[],\"Left\":[{\"id\":\"A\",\"label\":\"A\",\"type\":\"foundation.thermal_liquid.thermal_liquid\"}],\"Right\":[{\"id\":\"B\",\"label\":\"B\",\"type\":\"foundation.thermal_liquid.thermal_liquid\"}],\"Top\":[{\"id\":\"Na\",\"label\":\"Na\",\"type\":\"input\"},{\"id\":\"Nb\",\"label\":\"Nb\",\"type\":\"input\"}]}"
  "Flow Multiplier " : datacenter_lib/Flow Multiplier
      settings: InternalSimscapePortConfiguration="{\"Bottom\":[],\"Left\":[{\"id\":\"A\",\"label\":\"A\",\"type\":\"foundation.thermal_liquid.thermal_liquid\"}],\"Right\":[{\"id\":\"B\",\"label\":\"B\",\"type\":\"foundation.thermal_liquid.thermal_liquid\"}],\"Top\":[{\"id\":\"Na\",\"label\":\"Na\",\"type\":\"input\"},{\"id\":\"Nb\",\"label\":\"Nb\",\"type\":\"input\"}]}"
  Flow Rate Sensor (TL) : fl_lib/Thermal Liquid/Sensors/Flow Rate Sensor (TL)  mass_flow_measure=false  volumetric_flow_measure=true  energy_flow_measure=false
      settings: InternalSimscapePortConfiguration="{\"Bottom\":[],\"Left\":[{\"id\":\"A\",\"label\":\"A\",\"type\":\"foundation.thermal_liquid.thermal_liquid\"}],\"Right\":[{\"id\":\"B\",\"label\":\"B\",\"type\":\"foundation.thermal_liquid.thermal_liquid\"},{\"id\":\"V\",\"label\":\"V\",\"type\":\"output\"}],\"Top\":[]}"
  Flow Resistance (TL) : fl_lib/Thermal Liquid/Elements/Flow Resistance (TL)  delta_p_nominal=0.1*min(intFluidPrDrop) kPa  mdot_nominal=min(intFluidMdot) kg/s  area=intFluidPipeArea m^2  laminar_fraction=1e-3
  "Flow Resistance (TL) " : fl_lib/Thermal Liquid/Elements/Flow Resistance (TL)  delta_p_nominal=0.1*min(intFluidPrDrop) kPa  mdot_nominal=min(intFluidMdot) kg/s  area=intFluidPipeArea m^2  laminar_fraction=1e-3
  "Flow Resistance (TL)  " : fl_lib/Thermal Liquid/Elements/Flow Resistance (TL)  delta_p_nominal=0.1*min(intFluidPrDrop) kPa  mdot_nominal=min(intFluidMdot) kg/s  area=intFluidPipeArea m^2  laminar_fraction=1e-3
  InternalFluid : SimscapeFluids_lib/Thermal Liquid/Utilities/Thermal Liquid Properties (TL)  fluid_list=fluids.thermal_liquid.utilities.enum.thermal_liquid_fluid_list.water  concentration_param_EG=fluids.thermal_liquid.utilities.enum.thermal_liquid_concentration.volume_fraction  concentration_param_PG=fluids.thermal_liquid.utilities.enum.thermal_liquid_concentration.volume_fraction  c_mass_SW=3.5e-3  c_mass_EG=0.1  c_mass_PG=0.1  c_mass_GL=0.1  c_vol_EG=0.1  c_vol_PG=0.1  beta_const_EG=2.1791 GPa  beta_const_PG=2.1791 GPa  beta_const_GL=2.1791 GPa  p_min_EG=0.01 MPa  p_min_PG=0.01 MPa  p_min_GL=0.01 MPa  p_max_EG=50 MPa  p_max_PG=50 MPa  p_max_GL=50 MPa  p_atm=0.101325 MPa  properties_range_check=simscape.enum.assert.action.error
  One : fl_lib/Physical Signals/Sources/PS Constant  constant=1
  PS Saturation : fl_lib/Physical Signals/Nonlinear Operators/PS Saturation  upper_limit=speedLimFactor  lower_limit=0  ZeroCross=true
  Perfect Insulator1 : fl_lib/Thermal/Thermal Elements/Perfect Insulator  T_specify=off  T_priority=None  T=293.15 K  T_nominal_specify=off  T_nominal_value=1  T_nominal_unit=K
  Pressure & Temperature Sensor (TL) : fl_lib/Thermal Liquid/Sensors/Pressure & Temperature Sensor (TL)  reference=foundation.enum.MeasurementReference.difference  pressure=true  pressure_spec=foundation.enum.PressureMeasementSpec.Absolute  temperature=false
      settings: InternalSimscapePortConfiguration="{\"Bottom\":[],\"Left\":[{\"id\":\"A\",\"label\":\"A\",\"type\":\"foundation.thermal_liquid.thermal_liquid\"}],\"Right\":[{\"id\":\"B\",\"label\":\"B\",\"type\":\"foundation.thermal_liquid.thermal_liquid\"},{\"id\":\"P\",\"label\":\"P\",\"type\":\"output\"}],\"Top\":[]}"
  Pump Efficiency : datacenterCompositeLib/CDU (TL)/Pump Efficiency  SystemSampleTime=-1  VariantActivationTime=update diagram  EmptyChoice=off  PassThrough=off  PassThroughVariantControl=(default)  EmptyChoiceVariantControl=(default)  AllowFlexibleInterface=on  Latency=0  AutoFrameSizeCalculation=off
      settings: PortSchema="{\"entries\":[{\"content\":{\"sides\":[{\"content\":{\"connectorIds\":[\"LConn1\"]},\"type\":\"ConnectorPlacement.EquallySpacedRectSide\",\"uuid\":\"7c880f53-79d7-4fc1-b853-6a19eeb267d6\"},{\"content\":{\"connectorIds\":[\"RConn1\"],\"side\":\"RIGHT\"},\"type\":\"ConnectorPlacement.EquallySpacedRectSide\",\"uuid\":\"ee796b5d-8f71-4c2c-8982-d65c9b09dfff\"},{\"content\":{\"connectorIds\":[\"LConn2\",\"LConn3\"],\"side\":\"TOP\"},\"type\":\"ConnectorPlacement.EquallySpacedRectSide\",\"uuid\":\"11e8f51e-a30e-473a-bd43-abeec225f5c9\"}]},\"type\":\"ConnectorPlacement.EquallySpacedConnector\",\"uuid\":\"3106b96b-5b56-4bfa-809a-5c3e3f25fbb5\"}],\"packageUris\":[\"http://schema.mathworks.com/mf0/Connector/R2020b\"],\"version\":\"1.0\"}"
  Pump Nominal Rating : fl_lib/Physical Signals/Functions/PS Gain  gain=pumpNominalRPM rpm
  Specific Dissipation Heat Exchanger (TL-TL) : SimscapeFluids_lib/Heat Exchangers/Thermal Liquid/Specific Dissipation Heat Exchanger (TL-TL)  mdot1_TLU=intFluidMdot kg/s  mdot2_TLU=extFluidMdot kg/s  SD_TLU=spDissipationTbl kW/K  Q_check=simscape.enum.assert.action.none  mdot_dp_TLU_1=intFluidMdot kg/s  p_diff_TLU_1=intFluidPrDrop-0.3*min(intFluidPrDrop) kPa  T_ref_in_1=refT K  p_ref_in_1=refP MPa  mdot_threshold_1=1e-3 kg/s  liquid_volume_1=intFluidVol m^3  area_1=intFluidPipeArea m^2  mdot_dp_TLU_2=extFluidMdot kg/s  p_diff_TLU_2=extFluidPrDrop kPa  T_ref_in_2=refT K  p_ref_in_2=refP MPa  mdot_threshold_2=1e-3 kg/s  liquid_volume_2=extFluidVol m^3  area_2=extFluidPipeArea m^2  dynamic_compressibility_1=true  T0_1=iniT K  p0_1=iniP MPa  T_nominal_1=293.15 K  p_nominal_1=0.101325 MPa  dynamic_compressibility_2=true  T0_2=iniT K  p0_2=iniP MPa  T_nominal_2=293.15 K  p_nominal_2=0.101325 MPa
      settings: InternalSimscapePortConfiguration="{\"Bottom\":[],\"Left\":[{\"id\":\"A1\",\"label\":\"A1\",\"type\":\"foundation.thermal_liquid.thermal_liquid\"},{\"id\":\"B1\",\"label\":\"B1\",\"type\":\"foundation.thermal_liquid.thermal_liquid\"}],\"Right\":[{\"id\":\"A2\",\"label\":\"A2\",\"type\":\"foundation.thermal_liquid.thermal_liquid\"},{\"id\":\"B2\",\"label\":\"B2\",\"type\":\"foundation.thermal_liquid.thermal_liquid\"}],\"Top\":[]}"
  Subsystem : datacenterCompositeLib/CDU (TL)/Subsystem  SystemSampleTime=-1  VariantActivationTime=update diagram  EmptyChoice=off  PassThrough=off  PassThroughVariantControl=(default)  EmptyChoiceVariantControl=(default)  AllowFlexibleInterface=on  Latency=0  AutoFrameSizeCalculation=off
  numPump : fl_lib/Physical Signals/Nonlinear Operators/PS Saturation  upper_limit=nPumps  lower_limit=0  ZeroCross=true
  S : PMIOPort  Side=Left
  N : PMIOPort  Port=2  Side=Left
  Ae : PMIOPort  Port=3  Side=Left
  Ac : PMIOPort  Port=4  Side=Left
  Bc : PMIOPort  Port=5  Side=Left
  P : PMIOPort  Port=6  Side=Right
  Be : PMIOPort  Port=7  Side=Right
  connections:
  PS Saturation/LConn1 -- S/RConn1
  N/RConn1 -- numPump/LConn1
  Bc/RConn1 -- "Flow Resistance (TL)  "/LConn1
  Flow Multiplier/RConn1 -- Centrifugal Pump (TL)/LConn1
  Flow Rate Sensor (TL)/RConn2 -- Pump Efficiency/LConn2
  Centrifugal Pump (TL)/LConn2 -- "Flow Multiplier "/LConn1
  Pump Nominal Rating/RConn1 -- Subsystem/RConn1
  Pump Efficiency/LConn1 -- Pressure & Temperature Sensor (TL)/RConn2
  Pump Nominal Rating/LConn1 -- PS Saturation/RConn1
  P/RConn1 -- Pump Efficiency/RConn1
  "Flow Resistance (TL) "/RConn1 -- Specific Dissipation Heat Exchanger (TL-TL)/LConn1
  Flow Rate Sensor (TL)/RConn1 -- "Flow Multiplier "/RConn1
  Ae/RConn1 -- Specific Dissipation Heat Exchanger (TL-TL)/RConn1
  Centrifugal Pump (TL)/RConn1 -- Subsystem/LConn1
  Centrifugal Pump (TL)/RConn2 -- Subsystem/LConn2
  Be/RConn1 -- Specific Dissipation Heat Exchanger (TL-TL)/RConn2
  Perfect Insulator1/LConn1 -- Expansion Tank/RConn2
  Expansion Tank/RConn1 -- Ac/RConn1 -- Flow Resistance (TL)/LConn1
  Pressure & Temperature Sensor (TL)/LConn1 -- "Flow Resistance (TL)  "/RConn1 -- Flow Multiplier/LConn1
  "Flow Multiplier "/LConn3 -- Flow Multiplier/LConn2 -- One/RConn1
  InternalFluid/RConn1 -- Specific Dissipation Heat Exchanger (TL-TL)/LConn2 -- Flow Resistance (TL)/RConn1
  Flow Multiplier/LConn3 -- "Flow Multiplier "/LConn2 -- Pump Efficiency/LConn3 -- numPump/RConn1
  Flow Rate Sensor (TL)/LConn1 -- "Flow Resistance (TL) "/LConn1 -- Pressure & Temperature Sensor (TL)/RConn1

== system SimscapeCustomComponents_lib/Datacenter/Assemblies/PDU + CDU Assembly (TL-TL)/PDU Racks (TL) ==
  FMamb : datacenter_lib/Flow Multiplier
      settings: InternalSimscapePortConfiguration="{\"Bottom\":[],\"Left\":[{\"id\":\"A\",\"label\":\"A\",\"type\":\"foundation.thermal_liquid.thermal_liquid\"}],\"Right\":[{\"id\":\"B\",\"label\":\"B\",\"type\":\"foundation.thermal_liquid.thermal_liquid\"}],\"Top\":[{\"id\":\"Na\",\"label\":\"Na\",\"type\":\"input\"},{\"id\":\"Nb\",\"label\":\"Nb\",\"type\":\"input\"}]}"
  FMcdu : datacenter_lib/Flow Multiplier
      settings: InternalSimscapePortConfiguration="{\"Bottom\":[],\"Left\":[{\"id\":\"A\",\"label\":\"A\",\"type\":\"foundation.thermal_liquid.thermal_liquid\"}],\"Right\":[{\"id\":\"B\",\"label\":\"B\",\"type\":\"foundation.thermal_liquid.thermal_liquid\"}],\"Top\":[{\"id\":\"Na\",\"label\":\"Na\",\"type\":\"input\"},{\"id\":\"Nb\",\"label\":\"Nb\",\"type\":\"input\"}]}"
  PS Product : fl_lib/Physical Signals/Functions/PS Product
  Server Tray (TL) : Subsystem  mask{nGPU=nGPU, gpuTDPperDie=gpuTDPperDie, gpuIdlePower=gpuIdlePower, gpuHBMpower=gpuHBMpower, gpuExponent=gpuExponent, gpuHBMutil=gpuHBMutil, gpuLeakage=gpuLeakage, gpuNominalDieT=gpuNominalDieT, gpuDieThermalC=gpuDieThermalC, gpuHeatSinkR=gpuHeatSinkR, gpuSurfArea=gpuSurfArea, gpuAmbientR=gpuAmbientR, nCPU=nCPU, cpuTDPperSocket=cpuTDPperSocket, cpuIdlePower=cpuIdlePower, cpuExponent=cpuExponent, cpuLeakage=cpuLeakage, cpuNominalDieT=cpuNominalDieT, cpuDieThermalC=cpuDieThermalC, cpuHeatSinkR=cpuHeatSinkR, cpuSurfArea=cpuSurfArea, cpuAmbientR=cpuAmbientR, trayMass=trayMass, trayCp=trayCp, trayThermalR=trayThermalR, pipeLen=pipeLen, pipeArea=pipeArea, pipeDia=pipeDia, pipeLenXtra=pipeLenXtra, thermalKtc=thermalKtc, initialT=initialT, initialP=initialP, htc=htc}
      mask prompts: nGPU "Number of GPU (-)"; gpuTDPperDie "GPU TDP per die (W)"; gpuIdlePower "GPU idle power (W)"; gpuHBMpower "HBM power per GPU (W)"; gpuExponent "GPU power utilization exponent (-)"; gpuHBMutil "HBM utilization as fraction of compute utilization (-)"; gpuLeakage "Leakage increase per K above nominal temperature (W/K)"; gpuNominalDieT "Nominal die temperature at TDP (K)"; gpuDieThermalC "GPU die thermal capacitance (J/K)"; gpuHeatSinkR "GPU die-heat-sink thermal resistance (K/W)"; gpuSurfArea "Surface area per die for ambient heat transfer (m^2)"; gpuAmbientR "GPU die-ambient thermal resistance (K/W)"; nCPU "Number of CPU (-)"; cpuTDPperSocket "CPU TDP per socket (W)"; cpuIdlePower "CPU idle power per socket (W)"; cpuExponent "CPU power utilization exponent (-)"; cpuLeakage "Leakage increase per K above nominal temperature (W/K)"; cpuNominalDieT "Nominal die temperature at TDP (K)"; cpuDieThermalC "CPU die thermal capacitance (J/K)"; cpuHeatSinkR "CPU die-heat-sink thermal resistance (K/W)"; cpuSurfArea "Surface area per die for ambient heat transfer (m^2)"; cpuAmbientR "CPU die-ambient thermal resistance (K/W)"; trayMass "Tray mass (kg)"; trayCp "Tray specific heat capacity (J/kg*K)"; trayThermalR "Tray to external thermal resistance (K/W)"; pipeLen "Cold plate pipe length (m)"; pipeArea "Cold plate pipe cross-sectional area (m^2)"; pipeDia "Cold plate pipe hydraulic diameter (m)"; pipeLenXtra "Cold plate pipe aggregate equivalent length of local resistances (m)"; thermalKtc "Tray to cold plate thermal resistance (K/W)"; initialT "Initial temperature (K)"; initialP "Initial pressure (MPa)"; htc "Heat transfer coefficient to ambient (W/m^2.K)"
      settings: CopyFcn=set_param(gcbh,'LinkStatus','none');  PortSchema="{\"entries\":[{\"content\":{\"sides\":[{\"content\":{\"connectorIds\":[\"LConn1\",\"LConn2\",\"LConn3\"]},\"type\":\"ConnectorPlacement.EquallySpacedRectSide\",\"uuid\":\"d077d73c-67b3-4833-87c7-90e0b4257578\"},{\"content\":{\"connectorIds\":[\"RConn1\",\"RConn2\",\"RConn3\"],\"side\":\"RIGHT\"},\"type\":\"ConnectorPlacement.EquallySpacedRectSide\",\"uuid\":\"5339be23-611e-4862-9a5e-dd4e1a595af9\"},{\"content\":{\"side\":\"TOP\"},\"type\":\"ConnectorPlacement.EquallySpacedRectSide\",\"uuid\":\"df4f00c7-722c-4787-b527-29bc4d99befa\"},{\"content\":{\"connectorIds\":[\"RConn4\",\"RConn5\"],\"side\":\"BOTTOM\"},\"type\":\"ConnectorPlacement.EquallySpacedRectSide\",\"uuid\":\"45f86463-19b5-41c3-bb79-cbbcfbdd4a59\"}]},\"type\":\"ConnectorPlacement.EquallySpacedConnector\",\"uuid\":\"da9ddc4c-7978-4ef3-ba33-dfd55a606f60\"}],\"packageUris\":[\"http://schema.mathworks.com/mf0/Connector/R2020b\"],\"version\":\"1.0\"}"
      mask Help: web("DocumentationServerTrayTL.html")
      mask DialogControl Container6 Prompt: GPU
      mask DialogControl Container7 Prompt: CPU
      mask DialogControl Container9 Prompt: IT Tray
      mask DialogControl Container8 Prompt: Initial Conditions
      mask Display: image('icon_serverPlateTL.png');
  TMamb : datacenter_lib/Thermal Multiplier
      settings: InternalSimscapePortConfiguration="{\"Bottom\":[],\"Left\":[{\"id\":\"A\",\"label\":\"A\",\"type\":\"foundation.thermal.thermal\"}],\"Right\":[{\"id\":\"B\",\"label\":\"B\",\"type\":\"foundation.thermal.thermal\"}],\"Top\":[{\"id\":\"Na\",\"label\":\"Na\",\"type\":\"input\"},{\"id\":\"Nb\",\"label\":\"Nb\",\"type\":\"input\"}]}"
  nTraysXnRacks : fl_lib/Physical Signals/Sources/PS Constant  constant=nTrays*nRacks
  one : fl_lib/Physical Signals/Sources/PS Constant  constant=1
  U_gpu : PMIOPort  Side=Left
  U_cpu : PMIOPort  Port=2  Side=Left
  Ha : PMIOPort  Port=3  Side=Left
  P : PMIOPort  Port=4  Side=Right
  T_gpu : PMIOPort  Port=5  Side=Right
  T_cpu : PMIOPort  Port=6  Side=Right
  A : PMIOPort  Port=7  Side=Right
  B : PMIOPort  Port=8  Side=Right
  connections:
  TMamb/LConn1 -- Ha/RConn1
  TMamb/RConn1 -- Server Tray (TL)/LConn3
  Server Tray (TL)/LConn1 -- U_gpu/RConn1
  PS Product/RConn1 -- P/RConn1
  FMamb/RConn1 -- A/RConn1
  FMcdu/RConn1 -- B/RConn1
  one/RConn1 -- TMamb/LConn2 -- FMcdu/LConn3 -- FMamb/LConn3
  nTraysXnRacks/RConn1 -- FMamb/LConn2 -- FMcdu/LConn2 -- TMamb/LConn3 -- PS Product/LConn1
  FMamb/LConn1 -- Server Tray (TL)/RConn4
  FMcdu/LConn1 -- Server Tray (TL)/RConn5
  Server Tray (TL)/RConn2 -- T_gpu/RConn1
  Server Tray (TL)/RConn3 -- T_cpu/RConn1
  Server Tray (TL)/LConn2 -- U_cpu/RConn1
  Server Tray (TL)/RConn1 -- PS Product/LConn2
